simulink model "inverter_switching_model"  (R2023b)
settings: Solver=ode23tb  StartTime=0.0  StopTime=0.2  MaxStep=1e-5  RelTol=1e-3
InitFcn:
  | % Phase 3 – Day 2 Baseline Parameters
  | % Bring-up baseline only. No optimisation implied.
  | 
  | fsw = 5000;
  | f1  = 50;
  | m   = 0.3;
libraries: spsCurrentMeasurementLib x3, spsSeriesRLCBranchLib x2, spsVoltageMeasurementLib x2, spsThreePhaseSeriesRLCBranchLib x1, spsDCVoltageSourceLib x1, spsGroundLib x1, sps_lib x1, simulink x1, spsUniversalBridgeLib x1
settings Model: Creator=hwma  LastModifiedBy=hwma

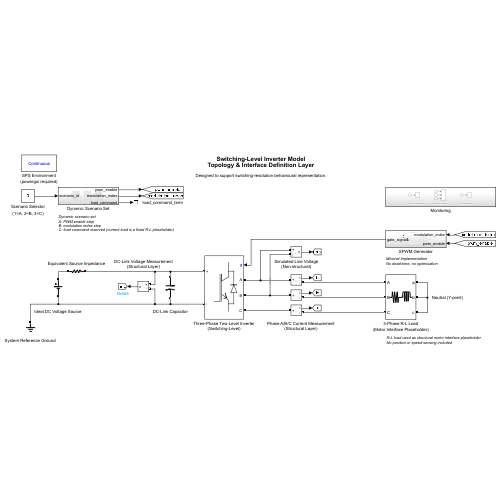
[thumbnail: Simulink's stored preview of the top-level diagram]
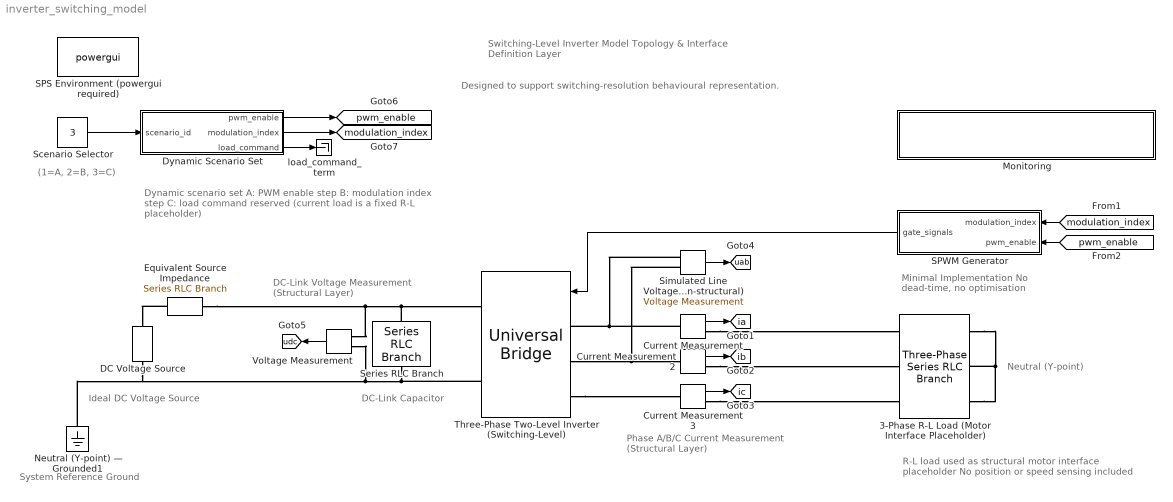
== system inverter_switching_model ==
  note: Minimal Implementation
      | No dead-time, no optimisation
  note: Phase A/B/C Current Measurement
      | (Structural Layer)
  note: DC-Link Capacitor
  note: Ideal DC Voltage Source
  note: Switching-Level Inverter Model
      | Topology & Interface Definition Layer
  note: System Reference Ground
  note: Neutral (Y-point)
  note: R-L load used as structural motor interface placeholder
      | No position or speed sensing included
  note: DC-Link Voltage Measurement
      | (Structural Layer)
  note: Designed to support switching-resolution behavioural representation.
  note: Dynamic scenario set
      | A: PWM enable step
      | B: modulation index step
      | C: load command reserved (current load is a fixed R-L placeholder)
  note: (1=A, 2=B, 3=C)
  3-Phase R-L Load (Motor Interface Placeholder) : spsThreePhaseSeriesRLCBranchLib/Three-Phase Series RLC Branch  LConnTagsString=A|B|C  RConnTagsString=A|B|C  BranchType=RL  Resistance=5  Inductance=0.005  Capacitance=1e-6  Measurements=None
  Current Measurement : spsCurrentMeasurementLib/Current Measurement  PhasorSimulation=off  OutputType=Complex  PSBequivalent=0
  Current Measurement2 : spsCurrentMeasurementLib/Current Measurement  PhasorSimulation=off  OutputType=Complex  PSBequivalent=0
  Current Measurement3 : spsCurrentMeasurementLib/Current Measurement  PhasorSimulation=off  OutputType=Complex  PSBequivalent=0
  DC Voltage Source : spsDCVoltageSourceLib/DC Voltage Source  Amplitude=400  Measurements=None
  Dynamic Scenario Set : Subsystem
  Equivalent Source Impedance : spsSeriesRLCBranchLib/Series RLC Branch  LConnTagsString=__new0  RConnTagsString=__new0  BranchType=R  Resistance=0.01  Inductance=1e-3  SetiL0=off  InitialCurrent=0  Capacitance=1e-6  Setx0=off  InitialVoltage=0  Measurements=None
  Monitoring : Subsystem
  Neutral (Y-point) — Grounded1 : spsGroundLib/Ground  LConnTagsString=a
  SPS Environment (powergui required) : sps_lib/powergui  Priority=1  SimulationMode=Continuous  SampleTime=50e-6  frequency=60  Iterations=50  frequencyindice=0  Pbase=100e6  ErrMax=1e-4  UnitsV=kV  UnitsW=MW  buscounter=0  FunctionMessages=off  echomessages=off  EnableUseOfTLC=off  CurrentSourceSwitches=off  DisableSnubberDevices=off  DisableRonSwitches=off  DisableVfSwitches=off  DisplayEquations=off  AutomaticDiscreteSolvers=off  SolverType=Tustin/Backward Euler (TBE)  Interpol=off  ExternalGateDelay=off  methode=off  Ts=100  x0status=blocks  SPID=on  SwTol=0  HookPort=off  NonlinearTolerance=1e-4  nMaxIteration=100  ContinueOnMaxIteration=off  RestoreLinks=warning  ResistiveCurrentMeasurement=off  Frange=[0:2:500]  Ylog=off  Xlog=on  ShowGrid=off  save=off  variable=ZData  structure=0  ZoomFFT=off  StartTime=0.0  cycles=1  DisplayStyle=1  fundamental=60  FreqAxis=off  MaxFrequency=1000  frequencyindicesteady=1  RmsSteady=1  display=off
  SPWM Generator : Subsystem
  Scenario Selector : Constant  Value=3  SampleTime=0
  Series RLC Branch : spsSeriesRLCBranchLib/Series RLC Branch  LConnTagsString=__new0  RConnTagsString=__new0  BranchType=C  Resistance=1  Inductance=1e-3  SetiL0=off  InitialCurrent=0  Capacitance=1e-3  Setx0=on  InitialVoltage=400  Measurements=None
  Simulated Line Voltage (Non-structural) : spsVoltageMeasurementLib/Voltage Measurement  PhasorSimulation=off  OutputType=Complex  PSBequivalent=0
  Three-Phase Two-Level Inverter (Switching-Level) : spsUniversalBridgeLib/Universal Bridge  Arms=3  SnubberResistance=1e5  SnubberCapacitance=1e-12  Device=IGBT / Diodes  Ron=1e-3  Lon=0  ForwardVoltages="[  0  0  ]"  ForwardVoltage=0  GTOparameters=[ 10e-6 , 20e-6 ]  IGBTparameters=[ 1e-6 , 2e-6 ]  Measurements=None  Measurements_2=None  converterType=Rectifier
  Voltage Measurement : spsVoltageMeasurementLib/Voltage Measurement  PhasorSimulation=off  OutputType=Complex  PSBequivalent=0
  load_command_term : Terminator
  tag scope: ia=global, ib=global, ic=global, modulation_index=global, pwm_enable=global, uab=global, udc=global
  wires:
  Current Measurement/1 -> [ia]
  Current Measurement2/1 -> [ib]
  Current Measurement3/1 -> [ic]
  Simulated Line Voltage (Non-structural)/1 -> [uab]
  SPWM Generator/1(gate_signals) -> Three-Phase Two-Level Inverter (Switching-Level)/1
  Voltage Measurement/1 -> [udc]
  Scenario Selector/1 -> Dynamic Scenario Set/1(scenario_id)
  Dynamic Scenario Set/1(pwm_enable) -> [pwm_enable]
  Dynamic Scenario Set/2(modulation_index) -> [modulation_index]
  Dynamic Scenario Set/3(load_command) -> load_command_term/1
  [modulation_index] -> SPWM Generator/1(modulation_index)
  [pwm_enable] -> SPWM Generator/2(pwm_enable)
  connections:
  3-Phase R-L Load (Motor Interface Placeholder)/RConn1 -- 3-Phase R-L Load (Motor Interface Placeholder)/RConn3 -- 3-Phase R-L Load (Motor Interface Placeholder)/RConn2
  Current Measurement/LConn1 -- Simulated Line Voltage (Non-structural)/LConn1 -- Three-Phase Two-Level Inverter (Switching-Level)/LConn1
  Current Measurement/RConn1 -- 3-Phase R-L Load (Motor Interface Placeholder)/LConn1
  Series RLC Branch/RConn1 -- Voltage Measurement/LConn2 -- Neutral (Y-point) — Grounded1/LConn1 -- DC Voltage Source/LConn1 -- Three-Phase Two-Level Inverter (Switching-Level)/RConn2
  Three-Phase Two-Level Inverter (Switching-Level)/LConn2 -- Simulated Line Voltage (Non-structural)/LConn2 -- Current Measurement2/LConn1
  Current Measurement2/RConn1 -- 3-Phase R-L Load (Motor Interface Placeholder)/LConn2
  Three-Phase Two-Level Inverter (Switching-Level)/LConn3 -- Current Measurement3/LConn1
  Current Measurement3/RConn1 -- 3-Phase R-L Load (Motor Interface Placeholder)/LConn3
  Equivalent Source Impedance/LConn1 -- Voltage Measurement/LConn1 -- Series RLC Branch/LConn1 -- Three-Phase Two-Level Inverter (Switching-Level)/RConn1
  Equivalent Source Impedance/RConn1 -- DC Voltage Source/RConn1

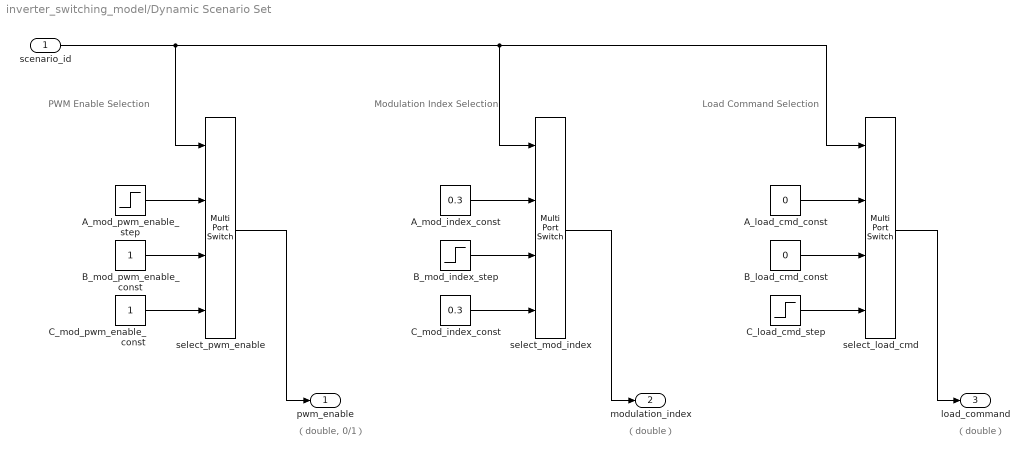
== system inverter_switching_model/Dynamic Scenario Set ==
  note: PWM Enable Selection
  note: （double）
  note: （double, 0/1）
  note: （double）
  note: Modulation Index Selection
  note: Load Command Selection
  scenario_id : Inport
  A_load_cmd_const : Constant  Value=0  SampleTime=0
  A_mod_index_const : Constant  Value=0.3  SampleTime=0
  A_mod_pwm_enable_step : Step  Time=0.05  SampleTime=0
  B_load_cmd_const : Constant  Value=0  SampleTime=0
  B_mod_index_step : Step  Time=0.05  Before=0.2  After=0.5  SampleTime=0
  B_mod_pwm_enable_const : Constant  SampleTime=0
  C_load_cmd_step : Step  Time=0.05  SampleTime=0
  C_mod_index_const : Constant  Value=0.3  SampleTime=0
  C_mod_pwm_enable_const : Constant  SampleTime=0
  select_load_cmd : MultiPortSwitch  DiagnosticForDefault=None  SaturateOnIntegerOverflow=off  InputSameDT=off
  select_mod_index : MultiPortSwitch  DiagnosticForDefault=None  SaturateOnIntegerOverflow=off  InputSameDT=off
  select_pwm_enable : MultiPortSwitch  DiagnosticForDefault=None  SaturateOnIntegerOverflow=off  InputSameDT=off
  pwm_enable : Outport
  modulation_index : Outport  Port=2
  load_command : Outport  Port=3
  wires:
  A_mod_pwm_enable_step/1 -> select_pwm_enable/2
  B_mod_pwm_enable_const/1 -> select_pwm_enable/3
  C_mod_pwm_enable_const/1 -> select_pwm_enable/4
  select_pwm_enable/1 -> pwm_enable/1
  select_mod_index/1 -> modulation_index/1
  C_mod_index_const/1 -> select_mod_index/4
  B_mod_index_step/1 -> select_mod_index/3
  A_mod_index_const/1 -> select_mod_index/2
  A_load_cmd_const/1 -> select_load_cmd/2
  B_load_cmd_const/1 -> select_load_cmd/3
  C_load_cmd_step/1 -> select_load_cmd/4
  select_load_cmd/1 -> load_command/1
  scenario_id/1 -> select_pwm_enable/1, select_mod_index/1, select_load_cmd/1

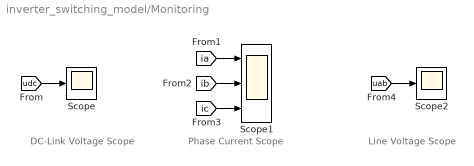
== system inverter_switching_model/Monitoring ==
  note: DC-Link Voltage Scope
  note: Phase Current Scope
  note: Line Voltage Scope
  Scope : Scope
  Scope1 : Scope  NumInputPorts=3
  Scope2 : Scope
  wires:
  [udc] -> Scope/1
  [ia] -> Scope1/1
  [ib] -> Scope1/2
  [ic] -> Scope1/3
  [uab] -> Scope2/1

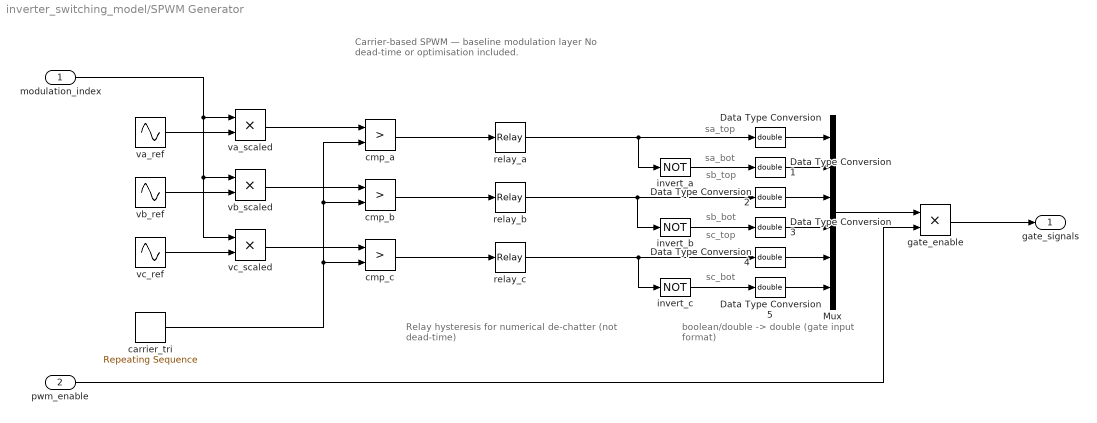
== system inverter_switching_model/SPWM Generator ==
  note: boolean/double -> double (gate input format)
  note: Carrier-based SPWM — baseline modulation layer
      | No dead-time or optimisation included.
  note: sa_top
  note: sa_bot
  note: sb_top
  note: sb_bot
  note: sc_top
  note: sc_bot
  note: Relay hysteresis for numerical de-chatter (not dead-time)
  modulation_index : Inport
  pwm_enable : Inport  Port=2
  Data Type Conversion{,1..5} (6 alike) : DataTypeConversion  OutDataTypeStr=double  SaturateOnIntegerOverflow=off  RndMeth=Floor
  Mux : Mux  Inputs=6
  carrier_tri : simulink/Sources/Repeating Sequence  rep_seq_t="[0  1/(2*fsw)  1/fsw]"  rep_seq_y="[-1  1  -1]"
  cmp_a : RelationalOperator  Operator=>  OutDataTypeStr=boolean  RndMeth=Simplest  InputSameDT=off
  cmp_b : RelationalOperator  Operator=>  OutDataTypeStr=boolean  RndMeth=Simplest  InputSameDT=off
  cmp_c : RelationalOperator  Operator=>  OutDataTypeStr=boolean  RndMeth=Simplest  InputSameDT=off
  gate_enable : Product
  invert_a : Logic  Operator=NOT  AllPortsSameDT=off  OutDataTypeStr=boolean
  invert_b : Logic  Operator=NOT  AllPortsSameDT=off  OutDataTypeStr=boolean
  invert_c : Logic  Operator=NOT  AllPortsSameDT=off  OutDataTypeStr=boolean
  relay_a : Relay  OnSwitchValue=+1e-6  OffSwitchValue=-1e-6
  relay_b : Relay  OnSwitchValue=+1e-6  OffSwitchValue=-1e-6
  relay_c : Relay  OnSwitchValue=+1e-6  OffSwitchValue=-1e-6
  va_ref : Sin  Frequency=2*pi*f1  SampleTime=0
  va_scaled : Product
  vb_ref : Sin  Frequency=2*pi*f1  Phase=-2*pi/3  SampleTime=0
  vb_scaled : Product
  vc_ref : Sin  Frequency=2*pi*f1  Phase=2*pi/3  SampleTime=0
  vc_scaled : Product
  gate_signals : Outport
  wires:
  Data Type Conversion2/1 -> Mux/3
  Data Type Conversion5/1 -> Mux/6
  Data Type Conversion/1 -> Mux/1
  Data Type Conversion4/1 -> Mux/5
  invert_c/1 -> Data Type Conversion5/1
  carrier_tri/1 -> cmp_c/2, cmp_b/2, cmp_a/2
  invert_a/1 -> Data Type Conversion1/1
  invert_b/1 -> Data Type Conversion3/1
  Data Type Conversion1/1 -> Mux/2
  Data Type Conversion3/1 -> Mux/4
  cmp_a/1 -> relay_a/1
  relay_a/1 -> invert_a/1, Data Type Conversion/1
  cmp_c/1 -> relay_c/1
  cmp_b/1 -> relay_b/1
  relay_b/1 -> invert_b/1, Data Type Conversion2/1
  relay_c/1 -> invert_c/1, Data Type Conversion4/1
  va_scaled/1 -> cmp_a/1
  va_ref/1 -> va_scaled/2
  vb_scaled/1 -> cmp_b/1
  vb_ref/1 -> vb_scaled/2
  vc_scaled/1 -> cmp_c/1
  vc_ref/1 -> vc_scaled/2
  modulation_index/1 -> va_scaled/1, vb_scaled/1, vc_scaled/1
  Mux/1 -> gate_enable/1
  gate_enable/1 -> gate_signals/1
  pwm_enable/1 -> gate_enable/2
